simulink model "Bicopter_Copy"  (R2025a)
settings: Solver=VariableStepAuto  StartTime=0.0  StopTime=10.0  RelTol=1e-3
values from neighbouring files (symbols this model uses):
  g = 9.81    [biCopter_Variable_script.m]
  initial_states = [initial_position; initial_angles; initial_velocity; initial_ang_velocity]    [biCopter_Variable_script.m]
  Ixx = 0.005    [biCopter_Variable_script.m]
  Iyy = 0.005    [biCopter_Variable_script.m]
  Izz = 0.01    [biCopter_Variable_script.m]
  k_T = 1.5e-6    (= 1.5e-06)    [biCopter_Variable_script.m]
  L = 0.25    [biCopter_Variable_script.m]
  m = 0.5    [biCopter_Variable_script.m]
  max_servo_angle = pi/6    (= 0.523598775598)    [biCopter_Variable_script.m]
  max_thrust_per_motor = 5    [biCopter_Variable_script.m]
  min_servo_angle = -pi/6    (= -0.523598775598)    [biCopter_Variable_script.m]
  min_thrust_per_motor = 0    [biCopter_Variable_script.m]
  tau_motor = 0.05    [biCopter_Variable_script.m]
undefined symbols (not defined in the file or in its folder): astar_path
libraries: rllib x1
settings Model: Creator=adity  LastModifiedBy=adity

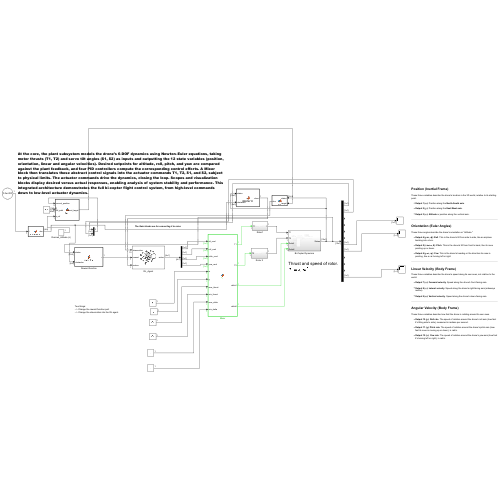
[thumbnail: Simulink's stored preview of the top-level diagram]
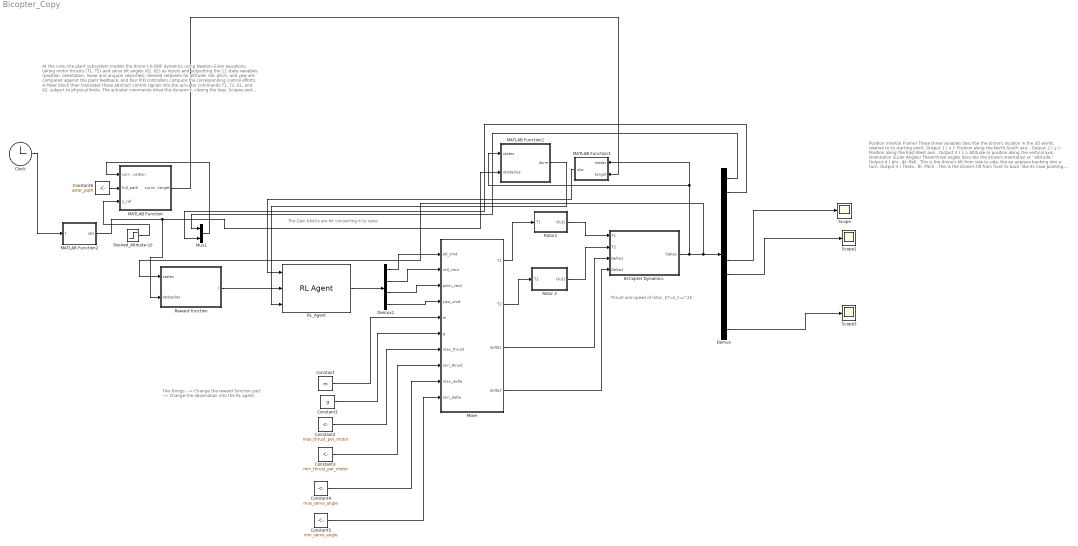
== system Bicopter_Copy ==
  note: Two things:
      | --> Change the reward function part
      | --> Change the observation into the RL agent.
  note: The Gain blocks are for converting it to rates
  note: Position (Inertial Frame)
      | These three variables describe the drone's location in the 3D world, relative to its starting point.
      | Output 1 ( x ): Position along the North-South axis .
      | Output 2 ( y ): Position along the East-West axis .
      | Output 3 ( z ): Altitude or position along the vertical axis.
      | Orientation (Euler Angles)
      | These three angles describe the drone's orientation or "attitude."
      | Output 4 ( phi , ϕ): Roll . This is the drone's tilt from side to side, like an airplane banking into a turn.
      | Output 5 ( theta , θ): Pitch . This is the drone's tilt from front to back, like its nose pointing up or down.
      | Output 6 ( psi , ψ): Yaw . This is the drone's heading or the direction its nose is pointing, like a car turning left or right.
      | Linear Velocity (Body Frame)
      | These three variables describe the drone's speed along its own axes, not relative to the world.
      | Output 7 ( u ): Forward velocity . Speed along the drone's front-facing axis.
      | Output 8 ( v ): Lateral velocity . Speed along the drone's right-facing axis (sideways motion).
      | Output 9 ( w ): Vertical velocity . Speed along the drone's down-facing axis.
      | Angular Velocity (Body Frame)
      | These three variables describe how fast the drone is rotating around its own axes.
      | Output 10 ( p ): Roll rate . The speed of rotation around the drone's roll axis (how fast it's tilting side to side), measured in radians per second.
      | Output 11 ( q ): Pitch rate . The speed of rotation around the drone's pitch axis (how fast its nose is moving up or down), in rad/s.
      | Output 12 ( r ): Yaw rate . The speed of rotation around the drone's yaw axis (how fast it's turning left or right), in rad/s.
  note: Thrust and speed of rotor.
      | $T=k_t​⋅ω^2$
  note: At the core, the plant subsystem models the drone’s 6-DOF dynamics using Newton–Euler equations, taking motor thrusts (T1, T2) and servo tilt angles (δ1, δ2) as inputs and outputting the 12 state variables (position, orientation, linear and angular velocities). Desired setpoints for altitude, roll, pitch, and yaw are compared against the plant feedback, and four PID controllers compute the corresponding control efforts. A Mixer block then translates these abstract control signals into the actuator commands T1, T2, δ1, and δ2, subject to physical limits. The actuator commands drive the dynamics, closing the loop. Scopes and visualization blocks display desired versus actual responses, enabling analysis of system stability and performance. This integrated architecture demonstrates the full bi-copter flight control system, from high-level commands down to low-level actuator dynamics.
  Bi-Copter Dynamics : Subsystem
  Clock : Clock
  Constant : Constant  Value=m
  Constant1 : Constant  Value=g
  Constant2 : Constant  Value=max_thrust_per_motor
  Constant3 : Constant  Value=min_thrust_per_motor
  Constant4 : Constant  Value=max_servo_angle
  Constant5 : Constant  Value=min_servo_angle
  Constant6 : Constant  Value=astar_path
  Demux : Demux  Outputs=12
  Demux1 : Demux
  Desired_Altitude (z) : Step  Time=0  After=500  SampleTime=0
  MATLAB Function : MATLAB Function  TreatAsAtomicUnit=on
  MATLAB Function1 : MATLAB Function  TreatAsAtomicUnit=on
  MATLAB Function2 : MATLAB Function  TreatAsAtomicUnit=on
  MATLAB Function3 : MATLAB Function  TreatAsAtomicUnit=on
  Mixer : MATLAB Function  TreatAsAtomicUnit=on
  Mux1 : Mux  Inputs=2
  RL_Agent : rllib/RL Agent  Agent=agentObj  ExternalActionAsInput=off  ProvideLastAction=off  ProvideCumRwd=off  TreatAsDirectFeedthrough=on  UseStrictObservationDataTypes=off
  Reward function : MATLAB Function  TreatAsAtomicUnit=on
  Rotor 2 : Subsystem
  Rotor1 : Subsystem
  Scope : Scope
      settings: ActiveDisplayYMinimum=-88.144858424605019  ActiveDisplayYMaximum=88.937365144154228
  Scope1 : Scope
      settings: ActiveDisplayYMinimum=-88.7441974939224  ActiveDisplayYMaximum=88.748617026885341
  Scope3 : Scope
      settings: ActiveDisplayYMinimum=-106.7500117856095  ActiveDisplayYMaximum=32.830412504409331  DataLoggingVariableName=ScopeData3
  wires:
  Desired_Altitude (z)/1 -> MATLAB Function/3(z_ref)
  Mixer/3(delta1) -> Bi-Copter Dynamics/3(Delta1)
  Mixer/4(delta2) -> Bi-Copter Dynamics/4(Delta2)
  Bi-Copter Dynamics/1(States) -> MATLAB Function3/1(states), MATLAB Function1/1(states), Reward function/1(states), Demux/1
  Constant/1 -> Mixer/5(m)
  Constant1/1 -> Mixer/6(g)
  Constant2/1 -> Mixer/7(max_thrust)
  Constant3/1 -> Mixer/8(min_thrust)
  Constant4/1 -> Mixer/9(max_delta)
  Constant5/1 -> Mixer/10(min_delta)
  Mixer/1(T1) -> Rotor1/1(T1)
  Rotor1/1(Out1) -> Bi-Copter Dynamics/1(T1)
  Mixer/2(T2) -> Rotor 2/1(T2)
  Rotor 2/1(Out1) -> Bi-Copter Dynamics/2(T2)
  Demux/7 -> Scope/1
  Demux/8 -> Scope1/1
  Demux/12 -> Scope3/1
  Demux/1 -> Mux1/1
  Demux/2 -> Mux1/2
  Mux1/1 -> MATLAB Function/1(current_position)
  Constant6/1 -> MATLAB Function/2(full_path)
  MATLAB Function/1(current_target) -> MATLAB Function3/2(target)
  Clock/1 -> MATLAB Function2/1(t)
  MATLAB Function2/1(obs) -> Reward function/2(obstacles), MATLAB Function1/2(obstacles)
  Demux1/1 -> Mixer/1(alt_cmd)
  Demux1/2 -> Mixer/2(roll_cmd)
  Demux1/3 -> Mixer/3(pitch_cmd)
  Demux1/4 -> Mixer/4(yaw_cmd)
  RL_Agent/1 -> Demux1/1
  MATLAB Function1/1(done) -> RL_Agent/3
  MATLAB Function3/1(obs) -> RL_Agent/1
  Reward function/1(r) -> RL_Agent/2

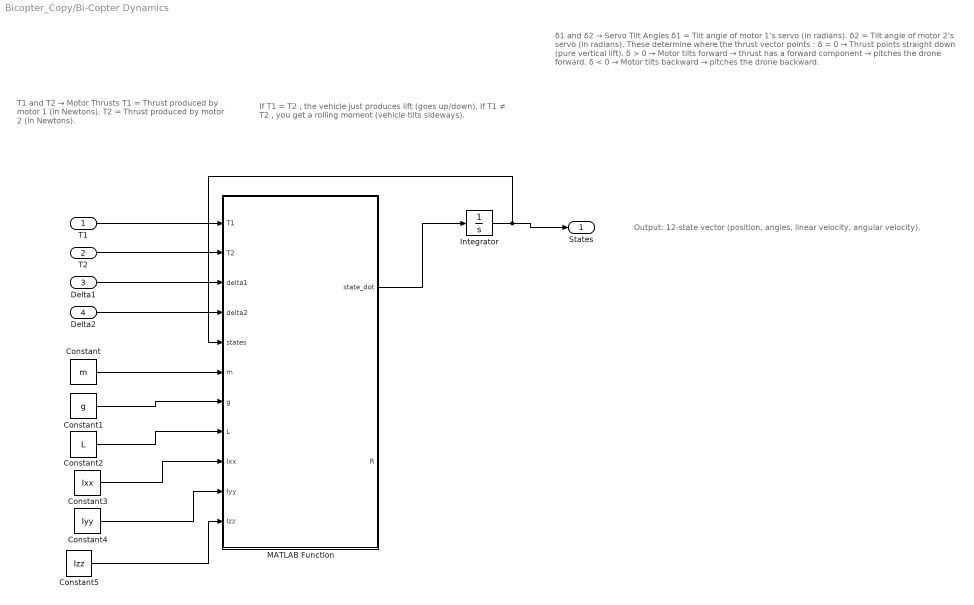
== system Bicopter_Copy/Bi-Copter Dynamics ==
  note: Output: 12-state vector (position, angles, linear velocity, angular velocity).
  note: δ1 and δ2 → Servo Tilt Angles
      | δ1 = Tilt angle of motor 1’s servo (in radians).
      | δ2 = Tilt angle of motor 2’s servo (in radians).
      | These determine where the thrust vector points :
      | δ = 0 → Thrust points straight down (pure vertical lift).
      | δ > 0 → Motor tilts forward → thrust has a forward component → pitches the drone forward.
      | δ < 0 → Motor tilts backward → pitches the drone backward.
  note: If T1 = T2 , the vehicle just produces lift (goes up/down).
      | If T1 ≠ T2 , you get a rolling moment (vehicle tilts sideways).
  note: T1 and T2 → Motor Thrusts
      | T1 = Thrust produced by motor 1 (in Newtons).
      | T2 = Thrust produced by motor 2 (in Newtons).
  T1 : Inport
  T2 : Inport  Port=2
  Delta1 : Inport  Port=3
  Delta2 : Inport  Port=4
  Constant : Constant  Value=m
  Constant1 : Constant  Value=g
  Constant2 : Constant  Value=L
  Constant3 : Constant  Value=Ixx
  Constant4 : Constant  Value=Iyy
  Constant5 : Constant  Value=Izz
  Integrator : Integrator  InitialCondition=initial_states
  MATLAB Function : MATLAB Function  TreatAsAtomicUnit=on
  States : Outport
  wires:
  MATLAB Function/1(state_dot) -> Integrator/1
  Integrator/1 -> MATLAB Function/5(states), States/1
  T1/1 -> MATLAB Function/1(T1)
  T2/1 -> MATLAB Function/2(T2)
  Delta1/1 -> MATLAB Function/3(delta1)
  Delta2/1 -> MATLAB Function/4(delta2)
  Constant/1 -> MATLAB Function/6(m)
  Constant1/1 -> MATLAB Function/7(g)
  Constant2/1 -> MATLAB Function/8(L)
  Constant3/1 -> MATLAB Function/9(Ixx)
  Constant4/1 -> MATLAB Function/10(Iyy)
  Constant5/1 -> MATLAB Function/11(Izz)

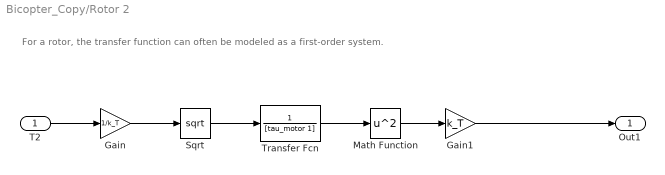
== system Bicopter_Copy/Rotor 2 ==
  note: For a rotor, the transfer function can often be modeled as a first-order system.
  T2 : Inport
  Gain : Gain  Gain=1/k_T
  Gain1 : Gain  Gain=k_T
  Math Function : Math  Operator=square
  Sqrt : Sqrt
  Transfer Fcn : TransferFcn  Denominator=[tau_motor 1]
  Out1 : Outport
  wires:
  T2/1 -> Gain/1
  Gain/1 -> Sqrt/1
  Sqrt/1 -> Transfer Fcn/1
  Transfer Fcn/1 -> Math Function/1
  Math Function/1 -> Gain1/1
  Gain1/1 -> Out1/1

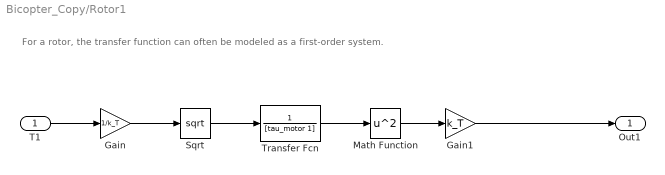
== system Bicopter_Copy/Rotor1 ==
  note: For a rotor, the transfer function can often be modeled as a first-order system.
  T1 : Inport
  Gain : Gain  Gain=1/k_T
  Gain1 : Gain  Gain=k_T
  Math Function : Math  Operator=square
  Sqrt : Sqrt
  Transfer Fcn : TransferFcn  Denominator=[tau_motor 1]
  Out1 : Outport
  wires:
  T1/1 -> Gain/1
  Gain/1 -> Sqrt/1
  Sqrt/1 -> Transfer Fcn/1
  Transfer Fcn/1 -> Math Function/1
  Math Function/1 -> Gain1/1
  Gain1/1 -> Out1/1

== matlab function Bicopter_Copy/Mixer ==
  data: alt_cmd input; T1 output; roll_cmd input; pitch_cmd input; yaw_cmd input; T2 output; delta1 output; delta2 output; m input; g input; max_thrust input; min_thrust input; max_delta input; min_delta input
function [T1, T2, delta1, delta2] = fcn(alt_cmd, roll_cmd, pitch_cmd, yaw_cmd, m, g, max_thrust, min_thrust, max_delta, min_delta)
base_thrust = m*g;
total_thrust = base_thrust + alt_cmd;
T1 = total_thrust/2 - roll_cmd;
T2 = total_thrust/2 + roll_cmd;
delta1 = pitch_cmd - yaw_cmd;
delta2 = pitch_cmd + yaw_cmd;
T1 = max(min_thrust, min(T1, max_thrust));
T2 = max(min_thrust, min(T2, max_thrust));
delta1 = max(min_delta, min(delta1, max_delta));
delta2 = max(min_delta, min(delta2, max_delta));
end

== matlab function Bicopter_Copy/Bi-Copter Dynamics/MATLAB Function ==
  data: T1 input; state_dot output; T2 input; delta1 input; delta2 input; states input; R output; m input; g input; L input; Ixx input; Iyy input; Izz input
function [state_dot, R] = fcn(T1, T2, delta1, delta2, states, m, g, L, Ixx, Iyy, Izz)
phi=states(4); theta=states(5); psi=states(6); 
u=states(7); v=states(8); w=states(9);
p=states(10); q=states(11); r=states(12);
cphi = cos(phi); sphi = sin(phi);
cthe = cos(theta); sthe = sin(theta);
cpsi = cos(psi); spsi = sin(psi);
R = [cthe*cpsi, sphi*sthe*cpsi-cphi*spsi, cphi*sthe*cpsi+sphi*spsi;
     cthe*spsi, sphi*sthe*spsi+cphi*cpsi, cphi*sthe*spsi-sphi*cpsi;
     -sthe,     sphi*cthe,              cphi*cthe];
Thrust_forces = [(T1*sin(delta1) + T2*sin(delta2));
                 0;
                 -(T1*cos(delta1) + T2*cos(delta2))];
Gravity_forces = R' * [0; 0; m*g];
uvw_dot = (1/m)*(Gravity_forces + Thrust_forces) - cross([p;q;r], [u;v;w]);
Torques = [L * (T1*cos(delta1) - T2*cos(delta2));
           L * (T1*sin(delta1) - T2*sin(delta2));
           L * (T1*sin(delta1) + T2*sin(delta2))]; 
pqr_dot = [1/Ixx; 1/Iyy; 1/Izz] .* (Torques - cross([p;q;r], [Ixx*p; Iyy*q; Izz*r]));
angle_dot = [1, sphi*tan(theta), cphi*tan(theta);
             0, cphi,            -sphi;
             0, sphi/cthe,       cphi/cthe] * [p;q;r];
pos_dot = R * [u;v;w];
state_dot = [pos_dot; angle_dot; uvw_dot; pqr_dot];
end

== matlab function Bicopter_Copy/MATLAB Function ==
  data: current_position input; current_target output; full_path input; z_ref input
function current_target = fcn(current_position, full_path, z_ref)
persistent path_waypoints;
persistent waypoint_index;
persistent num_waypoints;
if isempty(path_waypoints) || ~isequal(path_waypoints, full_path)
    path_waypoints = full_path;
    num_waypoints = size(path_waypoints, 1);
    waypoint_index = 1;
end
% Define a tolerance for reaching a waypoint (e.g., 0.5 meters)
REACHED_TOLERANCE = 0.5; 
% Get the current target waypoint coordinates
target_x = path_waypoints(waypoint_index, 1);
target_y = path_waypoints(waypoint_index, 2);
% Calculate the distance to the current target waypoint
dist_to_target = sqrt((current_position(1) - target_x)^2 + (current_position(2) - target_y)^2);
% If we are close enough to the current target, and it's not the final goal...
if (dist_to_target < REACHED_TOLERANCE) && (waypoint_index < num_waypoints)
    waypoint_index = waypoint_index + 1;
end
current_target_x = path_waypoints(waypoint_index, 1);
current_target_y = path_waypoints(waypoint_index, 2);
current_target = [current_target_x, current_target_y, z_ref];

end

== matlab function Bicopter_Copy/MATLAB Function1 ==
  data: states input; done output; obstacles input
function done = isDoneFcn(states, obstacles)
goal=[100 100 10];
x = states(1); y = states(2); z = states(3);
phi = states(4); theta = states(5);
maxTilt = deg2rad(60);
maxXY   = 50;   % since map = 100x100
minZ    = 0; 
maxZ    = 20;
done = 0;
if (abs(x) > maxXY) || (abs(y) > maxXY) || (z < minZ) || (z > maxZ)
    done = 1;
end
if abs(phi) > maxTilt || abs(theta) > maxTilt
    done = 1;
end
if norm([x - goal(1), y - goal(2), z - goal(3)]) < 2
    done = 1;
end
for i = 1:size(obstacles,1)
    if norm([x - obstacles(i,1), y - obstacles(i,2), z - obstacles(i,3)]) < 2
        done = 1;
    end
end
end

== matlab function Bicopter_Copy/MATLAB Function2 ==
  data: t input; obs output
function obs = obstaclesFcn(t)
    base = [20 20 0;   % Obstacle 1
            40 60 0;   % Obstacle 2
            70 30 0;   % Obstacle 3
            80 80 0];  % Obstacle 4
    amp = [10  0  0;   % Obs 1 moves along X
           0   5  0;   % Obs 2 moves along Y
           5   5  0;   % Obs 3 moves in diagonal (XY)
           0   0  2];  % Obs 4 moves up & down in Z
    freq = [0.1 0 0;
            0 0.2 0;
            0.15 0.15 0;
            0 0 0.3];
    N = size(base,1);
    obs = zeros(N,3);
    for i = 1:N
        obs(i,1) = base(i,1) + amp(i,1)*sin(freq(i,1)*t);
        obs(i,2) = base(i,2) + amp(i,2)*sin(freq(i,2)*t);
        obs(i,3) = base(i,3) + amp(i,3)*sin(freq(i,3)*t);
    end
end

== matlab function Bicopter_Copy/MATLAB Function3 ==
  data: states input; obs output; target input
function obs = fcn(states, target)
    x     = states(1); 
    y     = states(2); 
    z     = states(3);
    phi   = states(4); 
    theta = states(5); 
    psi   = states(6);
    u     = states(7); 
    v     = states(8); 
    w     = states(9);
    p     = states(10); 
    q     = states(11); 
    r     = states(12);
    x_ref = target(1); 
    y_ref = target(2); 
    z_ref = target(3);
    err_pos = [x_ref - x, y_ref - y, z_ref - z];
    yaw_err = atan2(sin(psi), cos(psi));
    obs = [err_pos, phi, theta, yaw_err, u, v, w, p, q, r];
end

== matlab function Bicopter_Copy/Reward function ==
  data: states input; r output; obstacles input
function r = rewardFcn(states, obstacles)
target=[100 100 10];
x = states(1); y = states(2); z = states(3);
u = states(7); v = states(8); w = states(9);
dist_to_target = norm([x - target(1), y - target(2), z - target(3)]);
r = -0.1 * dist_to_target;
r = r - 0.01 * norm([u, v, w]);
if dist_to_target < 2
    r = r + 100;
end
for i = 1:size(obstacles,1)
    if norm([x - obstacles(i,1), y - obstacles(i,2), z - obstacles(i,3)]) < 2
        r = r - 100;
    end
end
end
